simulink model "IM_drive_Simulink"  (R2018b)
settings: Solver=ode45  StartTime=0.0  StopTime=10.0  RelTol=1e-6  AbsTol=1e-8
values from neighbouring files (symbols this model uses):
  AntiW = 1    [IM_drive_main_code.m]
  B = 0.08    [IM_drive_main_code.m]
  Ba = (alfaw*Jhat-Bhat)*1    (= 0.17)    [IM_drive_main_code.m]
  Flux_ref = 0.9    [IM_drive_main_code.m]
  Flux_ref_time = 0.001    [IM_drive_main_code.m]
  invL_matrix = inv(LMAT)    [IM_drive_main_code.m]
  ir_alpha_0 = 0    [IM_drive_main_code.m]
  ir_beta_0 = 0    [IM_drive_main_code.m]
  is_alpha_0 = 0    [IM_drive_main_code.m]
  is_beta_0 = 0    [IM_drive_main_code.m]
  Israted = 9.1*sqrt(2)    [IM_drive_main_code.m]
  J = 0.0125    [IM_drive_main_code.m]
  Kic = alfac*(Rshat+RRhat+Ra)    (= 15552.4475524)    [IM_drive_main_code.m]
  Kiw = alfaw*(Bhat+Ba)    (= 5)    [IM_drive_main_code.m]
  Kpc = alfac*Lsigmahat    (= 15.5524475524)    [IM_drive_main_code.m]
  Kpw = alfaw*Jhat    (= 0.25)    [IM_drive_main_code.m]
  Lm = 0.135    [IM_drive_main_code.m]
  LMhat = LM*0.9    (= 0.114702797203)    [IM_drive_main_code.m]
  Lr = Lm+Lrl    (= 0.143)    [IM_drive_main_code.m]
  Lsigmahat = Lsigma*1    (= 0.0155524475524)    [IM_drive_main_code.m]
  np = 2    [IM_drive_main_code.m]
  PsiRhat0 = 0    [IM_drive_main_code.m]
  Ra = (alfac*Lsigmahat-Rshat-RRhat)*1    (= 13.1173079368)    [IM_drive_main_code.m]
  RR = (Lm/Lr)^2*Rr    (= 1.10513961563)    [IM_drive_main_code.m]
  Rr = 1.24    [IM_drive_main_code.m]
  RRhat = RR*1    (= 1.10513961563)    [IM_drive_main_code.m]
  Rs = 1.33    [IM_drive_main_code.m]
  Te_ref1 = 12    [IM_drive_main_code.m]
  Te_ref2 = 8    [IM_drive_main_code.m]
  Te_reftime1 = 1    [IM_drive_main_code.m]
  Te_reftime2 = 2    [IM_drive_main_code.m]
  Te_reftime3 = 2.1    [IM_drive_main_code.m]
  thetahat0 = 0    [IM_drive_main_code.m]
  thetar_0 = 0    [IM_drive_main_code.m]
  TL_extra = 14.6    [IM_drive_main_code.m]
  TL_extra_time = 10    [IM_drive_main_code.m]
  Umax = VconvLim    [IM_drive_main_code.m]
  VconvLim = 440*sqrt(2/3)    [IM_drive_main_code.m]
  wr_0 = 0    [IM_drive_main_code.m]
  Wr_ref_step = 1435*pi/30    (= 150.272848597)    [IM_drive_main_code.m]
  Wr_ref_step_time = 1.0    (= 1)    [IM_drive_main_code.m]
undefined symbols (not defined in the file or in its folder): j
settings Model: ExtModeTrigMode=oneshot  ExtModeArmWhenConnect=off  ExtModeAutoUpdateStatusClock=off  Creator=e6zebra  LastModifiedBy=e6zebra
settings SolverCC: AutoScaleAbsTol=off
settings DataIOCC: SaveFormat=Array  SignalLoggingSaveFormat=ModelDataLogs
settings OptimizationCC: BlockReduction=off  BooleanDataType=off  ExpressionDepthLimit=2147483647  InitFltsAndDblsToZero=on  LifeSpan=inf
settings DebuggingCC: SaveWithParameterizedLinksMsg=none  UnderspecifiedInitializationDetection=Classic  MergeDetectMultiDrivingBlocksExec=none  SignalResolutionControl=TryResolveAllWithWarning  MultiTaskDSMMsg=warning  MultiTaskCondExecSysMsg=none  FcnCallInpInsideContextMsg=warning  StateNameClashWarn=warning  SFUnexpectedBacktrackingDiag=warning  SFNoUnconditionalDefaultTransitionDiag=warning  SFExecutionAtInitializationDiag=none
settings HardwareCC: ProdBitPerPointer=32  ProdBitPerSizeT=32  ProdBitPerPtrDiffT=32  ProdLargestAtomicFloat=None  ProdIntDivRoundTo=Undefined  ProdEndianess=Unspecified  ProdWordSize=32  ProdHWDeviceType=32-bit Generic  TargetUnknown=on
settings ModelReferenceCC: PropagateSignalLabelsOutOfModel=off
settings SFSimCC: SimUseLocalCustomCode=off
settings RTWCC: TemplateMakefile=grt.tmf  RTWUseLocalCustomCode=off
settings CodeAppCC: StateflowObjectComments=on
settings GRTTargetCC: TargetFcnLib=ansi_tfl_tmw.mat  TargetLangStandard=C89/C90 (ANSI)  GeneratePreprocessorConditionals=Disable all  CombineOutputUpdateFcns=off  GRTInterface=on
settings ConfigComp: CovMetricSettings=dw  CovHtmlReporting=on  CovSaveCumulativeToWorkspaceVar=on  CovSaveSingleToWorkspaceVar=on  CovExternalEMLEnable=off

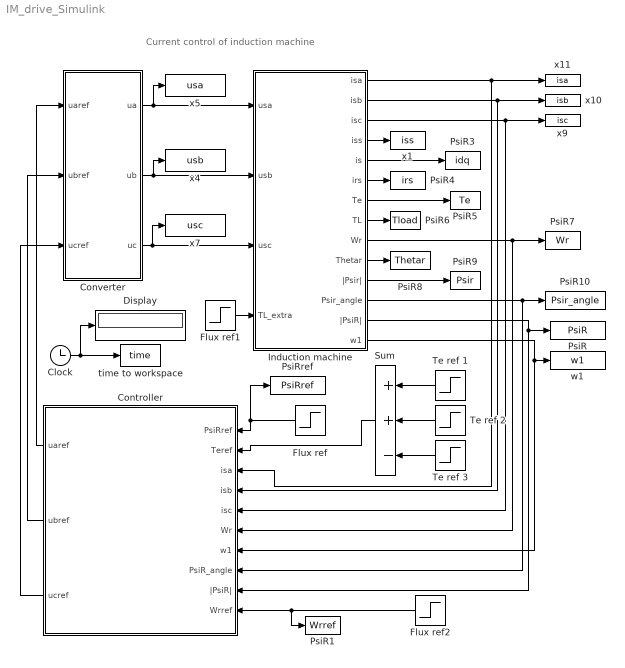
== system IM_drive_Simulink ==
  note: Current control of induction machine
  Clock : Clock
  Controller : Subsystem
  Converter : Subsystem
  Display : Display
  Flux ref : Step  Time=Flux_ref_time  After=Flux_ref  SampleTime=0
  Flux ref1 : Step  Time=TL_extra_time  After=TL_extra  SampleTime=0
  Flux ref2 : Step  Time=Wr_ref_step_time  After=Wr_ref_step  SampleTime=0
  Induction machine : Subsystem
  PsiR : ToWorkspace  VariableName=PsiR  SampleTime=-1
  PsiR1 : ToWorkspace  VariableName=Wrref  SampleTime=-1
  PsiR10 : ToWorkspace  VariableName=Psir_angle  SampleTime=-1
  PsiR3 : ToWorkspace  VariableName=idq  SampleTime=-1
  PsiR4 : ToWorkspace  VariableName=irs  SampleTime=-1
  PsiR5 : ToWorkspace  VariableName=Te  SampleTime=-1
  PsiR6 : ToWorkspace  VariableName=Tload  SampleTime=-1
  PsiR7 : ToWorkspace  VariableName=Wr  SampleTime=-1
  PsiR8 : ToWorkspace  VariableName=Thetar  SampleTime=-1
  PsiR9 : ToWorkspace  VariableName=Psir  SampleTime=-1
  PsiRref : ToWorkspace  VariableName=PsiRref  SampleTime=-1
  Sum : Sum  Inputs=++-  SaturateOnIntegerOverflow=on
  Te ref 1 : Step  Time=Te_reftime1  After=Te_ref1  SampleTime=0
  Te ref 2 : Step  Time=Te_reftime2  After=Te_ref2  SampleTime=0
  Te ref 3 : Step  Time=Te_reftime3  After=Te_ref2  SampleTime=0
  time to workspace : ToWorkspace  VariableName=time  SampleTime=-1
  w1 : ToWorkspace  VariableName=w1  SampleTime=-1
  x1 : ToWorkspace  VariableName=iss  SampleTime=-1
  x10 : ToWorkspace  VariableName=isb  SampleTime=-1
  x11 : ToWorkspace  VariableName=isa  SampleTime=-1
  x4 : ToWorkspace  VariableName=usb  SampleTime=-1
  x5 : ToWorkspace  VariableName=usa  SampleTime=-1
  x7 : ToWorkspace  VariableName=usc  SampleTime=-1
  x9 : ToWorkspace  VariableName=isc  SampleTime=-1
  wires:
  Clock/1 -> time to workspace/1, Display/1
  Te ref 1/1 -> Sum/1
  Te ref 3/1 -> Sum/3
  Te ref 2/1 -> Sum/2
  Converter/1(ua) -> Induction machine/1(usa), x5/1
  Converter/2(ub) -> Induction machine/2(usb), x4/1
  Converter/3(uc) -> x7/1, Induction machine/3(usc)
  Induction machine/4(iss) -> x1/1
  Induction machine/5(is) -> PsiR3/1
  Induction machine/7(Te) -> PsiR5/1
  Induction machine/6(irs) -> PsiR4/1
  Induction machine/9(Wr) -> Controller/6(Wr), PsiR7/1
  Induction machine/8(TL) -> PsiR6/1
  Induction machine/11(|Psir|) -> PsiR9/1
  Induction machine/10(Thetar) -> PsiR8/1
  Induction machine/12(Psir_angle) -> PsiR10/1, Controller/8(PsiR_angle)
  Induction machine/3(isc) -> Controller/5(isc), x9/1
  Induction machine/2(isb) -> Controller/4(isb), x10/1
  Induction machine/1(isa) -> x11/1, Controller/3(isa)
  Flux ref1/1 -> Induction machine/4(TL_extra)
  Induction machine/13(|PsiR|) -> Controller/9(|PsiR|), PsiR/1
  Induction machine/14(w1) -> Controller/7(w1), w1/1
  Flux ref/1 -> Controller/1(PsiRref), PsiRref/1
  Sum/1 -> Controller/2(Teref)
  Controller/1(uaref) -> Converter/1(uaref)
  Controller/2(ubref) -> Converter/2(ubref)
  Controller/3(ucref) -> Converter/3(ucref)
  Flux ref2/1 -> PsiR1/1, Controller/10(Wrref)

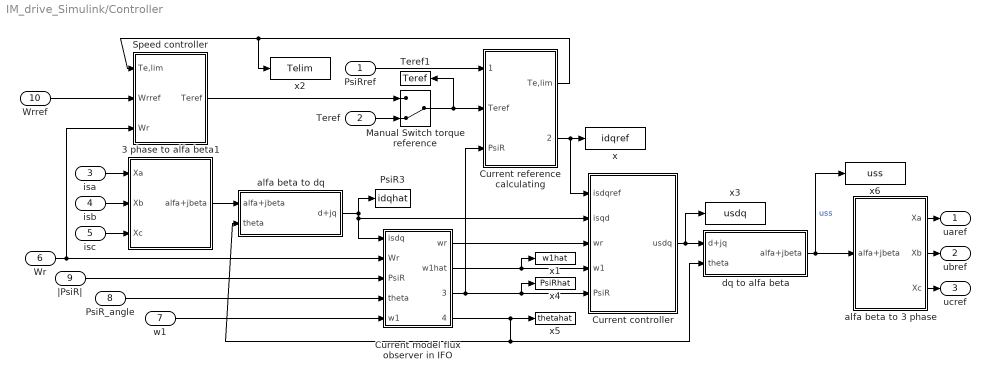
== system IM_drive_Simulink/Controller ==
  PsiRref : Inport
  Teref : Inport  Port=2
  isa : Inport  Port=3
  isb : Inport  Port=4
  isc : Inport  Port=5
  Wr : Inport  Port=6
  w1 : Inport  Port=7
  PsiR_angle : Inport  Port=8
  |PsiR| : Inport  Port=9
  Wrref : Inport  Port=10
  3 phase to alfa beta1 : Subsystem
  Current controller : Subsystem
  Current model flux observer in IFO : Subsystem
  Current reference calculating : Subsystem
  Manual Switch torque reference : ManualSwitch  CurrentSetting=0
  PsiR3 : ToWorkspace  VariableName=idqhat  SampleTime=-1
  Speed controller : Subsystem
  Teref1 : ToWorkspace  VariableName=Teref  SampleTime=-1
  alfa beta to 3 phase : Subsystem
  alfa beta to dq : Subsystem
  dq to alfa beta : Subsystem
  x : ToWorkspace  VariableName=idqref  SampleTime=-1
  x1 : ToWorkspace  VariableName=w1hat  SampleTime=-1
  x2 : ToWorkspace  VariableName=Telim  SampleTime=-1
  x3 : ToWorkspace  VariableName=usdq  SampleTime=-1
  x4 : ToWorkspace  VariableName=PsiRhat  SampleTime=-1
  x5 : ToWorkspace  VariableName=thetahat  SampleTime=-1
  x6 : ToWorkspace  VariableName=uss  SampleTime=-1
  uaref : Outport
  ubref : Outport  Port=2
  ucref : Outport  Port=3
  wires:
  PsiRref/1 -> Current reference calculating/1(PsiRref)
  alfa beta to 3 phase/1(Xa) -> uaref/1
  alfa beta to 3 phase/2(Xb) -> ubref/1
  alfa beta to 3 phase/3(Xc) -> ucref/1
  Current controller/1(usdq) -> x3/1, dq to alfa beta/1(d+jq)
  Current reference calculating/2(isdqref) -> Current controller/1(isdqref), x/1
  dq to alfa beta/1(alfa+jbeta) -> x6/1, alfa beta to 3 phase/1(alfa+jbeta)  "uss"
  Teref/1 -> Manual Switch torque reference/2
  Wr/1 -> Speed controller/3(Wr), Current model flux observer in IFO/2(Wr)
  alfa beta to dq/1(d+jq) -> Current controller/2(isqd), Current model flux observer in IFO/1(isdq), PsiR3/1
  3 phase to alfa beta1/1(alfa+jbeta) -> alfa beta to dq/1(alfa+jbeta)
  isa/1 -> 3 phase to alfa beta1/1(Xa)
  isc/1 -> 3 phase to alfa beta1/3(Xc)
  isb/1 -> 3 phase to alfa beta1/2(Xb)
  Manual Switch torque reference/1 -> Teref1/1, Current reference calculating/2(Teref)
  Current model flux observer in IFO/1(wr) -> Current controller/3(wr)
  Current model flux observer in IFO/2(w1hat) -> x1/1, Current controller/4(w1)
  Current model flux observer in IFO/3(PsiRhat) -> Current reference calculating/3(PsiR), x4/1, Current controller/5(PsiR)
  Current reference calculating/1(Te,lim) -> x2/1, Speed controller/1(Te,lim)
  Speed controller/1(Teref) -> Manual Switch torque reference/1
  w1/1 -> Current model flux observer in IFO/5(w1)
  |PsiR|/1 -> Current model flux observer in IFO/3(PsiR)
  PsiR_angle/1 -> Current model flux observer in IFO/4(theta)
  Current model flux observer in IFO/4(thetahat) -> dq to alfa beta/2(theta), alfa beta to dq/2(theta), x5/1
  Wrref/1 -> Speed controller/2(Wrref)

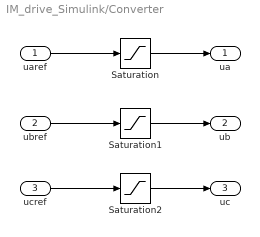
== system IM_drive_Simulink/Converter ==
  uaref : Inport
  ubref : Inport  Port=2
  ucref : Inport  Port=3
  Saturation : Saturate  UpperLimit=VconvLim  LowerLimit=-VconvLim
  Saturation1 : Saturate  UpperLimit=VconvLim  LowerLimit=-VconvLim
  Saturation2 : Saturate  UpperLimit=VconvLim  LowerLimit=-VconvLim
  ua : Outport
  ub : Outport  Port=2
  uc : Outport  Port=3
  wires:
  Saturation2/1 -> uc/1
  Saturation1/1 -> ub/1
  Saturation/1 -> ua/1
  uaref/1 -> Saturation/1
  ubref/1 -> Saturation1/1
  ucref/1 -> Saturation2/1

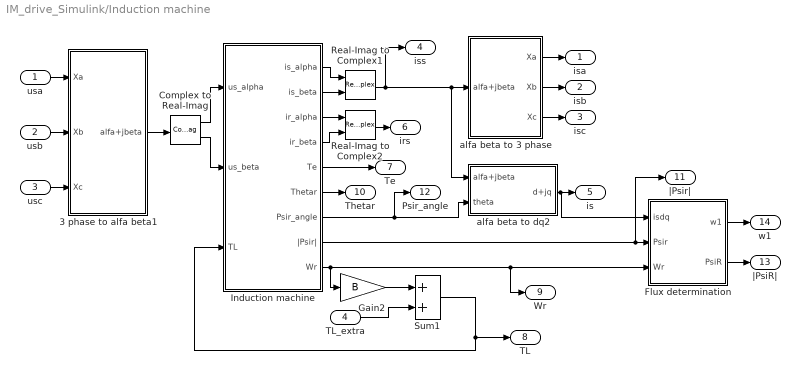
== system IM_drive_Simulink/Induction machine ==
  usa : Inport
  usb : Inport  Port=2
  usc : Inport  Port=3
  TL_extra : Inport  Port=4
  3 phase to alfa beta1 : Subsystem
  Complex to Real-Imag : ComplexToRealImag
  Flux determination : Subsystem
  Gain2 : Gain  Gain=B
  Induction machine : Subsystem
  Real-Imag to Complex1 : RealImagToComplex
  Real-Imag to Complex2 : RealImagToComplex
  Sum1 : Sum  SaturateOnIntegerOverflow=on  InputSameDT=on  OutDataTypeStr=Inherit: Same as first input
  alfa beta to 3 phase : Subsystem
  alfa beta to dq2 : Subsystem
  isa : Outport
  isb : Outport  Port=2
  isc : Outport  Port=3
  iss : Outport  Port=4
  is : Outport  Port=5
  irs : Outport  Port=6
  Te : Outport  Port=7
  TL : Outport  Port=8
  Wr : Outport  Port=9
  Thetar : Outport  Port=10
  |Psir| : Outport  Port=11
  Psir_angle : Outport  Port=12
  |PsiR| : Outport  Port=13
  w1 : Outport  Port=14
  wires:
  TL_extra/1 -> Sum1/2
  Real-Imag to Complex1/1 -> iss/1, alfa beta to 3 phase/1(alfa+jbeta), alfa beta to dq2/1(alfa+jbeta)
  alfa beta to dq2/1(d+jq) -> Flux determination/1(isdq), is/1
  Real-Imag to Complex2/1 -> irs/1
  Sum1/1 -> Induction machine/3(TL), TL/1
  Gain2/1 -> Sum1/1
  3 phase to alfa beta1/1(alfa+jbeta) -> Complex to Real-Imag/1
  usc/1 -> 3 phase to alfa beta1/3(Xc)
  usb/1 -> 3 phase to alfa beta1/2(Xb)
  usa/1 -> 3 phase to alfa beta1/1(Xa)
  alfa beta to 3 phase/1(Xa) -> isa/1
  alfa beta to 3 phase/3(Xc) -> isc/1
  alfa beta to 3 phase/2(Xb) -> isb/1
  Flux determination/2(PsiR) -> |PsiR|/1
  Flux determination/1(w1) -> w1/1
  Induction machine/7(Psir_angle) -> alfa beta to dq2/2(theta), Psir_angle/1
  Induction machine/9(Wr) -> Wr/1, Flux determination/3(Wr), Gain2/1
  Complex to Real-Imag/1 -> Induction machine/1(us_alpha)
  Complex to Real-Imag/2 -> Induction machine/2(us_beta)
  Induction machine/1(is_alpha) -> Real-Imag to Complex1/1
  Induction machine/2(is_beta) -> Real-Imag to Complex1/2
  Induction machine/3(ir_alpha) -> Real-Imag to Complex2/1
  Induction machine/4(ir_beta) -> Real-Imag to Complex2/2
  Induction machine/5(Te) -> Te/1
  Induction machine/6(Thetar) -> Thetar/1
  Induction machine/8(|Psir|) -> |Psir|/1, Flux determination/2(Psir)

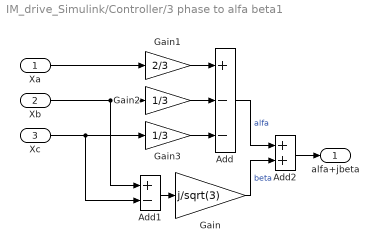
== system IM_drive_Simulink/Controller/3 phase to alfa beta1 ==
  Xa : Inport
  Xb : Inport  Port=2
  Xc : Inport  Port=3
  Add : Sum  Inputs=+--
  Add1 : Sum  Inputs=+-
  Add2 : Sum
  Gain : Gain  Gain=j/sqrt(3)
  Gain1 : Gain  Gain=2/3
  Gain2 : Gain  Gain=1/3
  Gain3 : Gain  Gain=1/3
  alfa+jbeta : Outport
  wires:
  Add1/1 -> Gain/1
  Add2/1 -> alfa+jbeta/1
  Gain/1 -> Add2/2  "beta"
  Add/1 -> Add2/1  "alfa"
  Gain3/1 -> Add/3
  Gain2/1 -> Add/2
  Gain1/1 -> Add/1
  Xa/1 -> Gain1/1
  Xb/1 -> Gain2/1, Add1/1
  Xc/1 -> Gain3/1, Add1/2

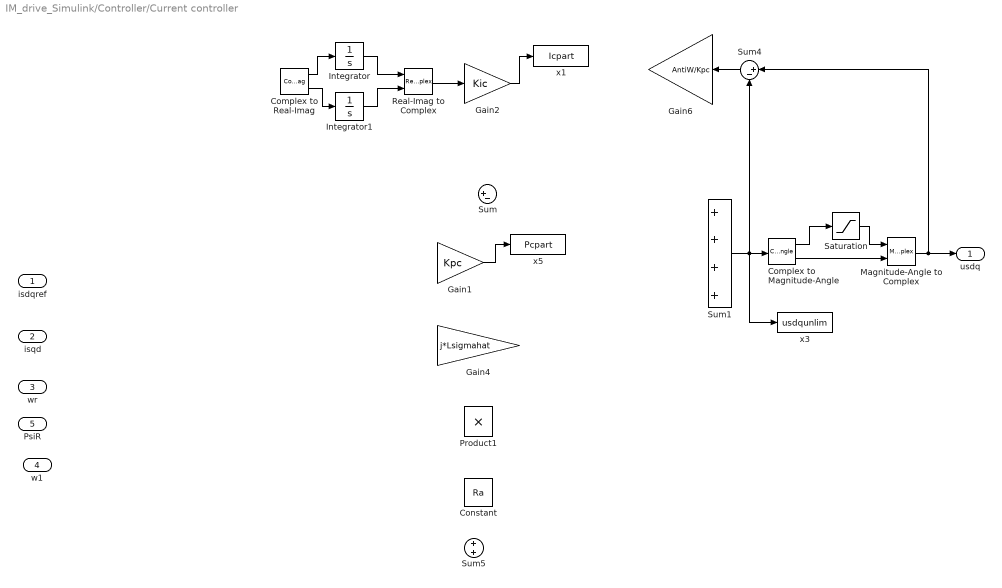
== system IM_drive_Simulink/Controller/Current controller ==
  isdqref : Inport
  isqd : Inport  Port=2
  wr : Inport  Port=3
  w1 : Inport  Port=4
  PsiR : Inport  Port=5
  Complex to Magnitude-Angle : ComplexToMagnitudeAngle
  Complex to Real-Imag : ComplexToRealImag
  Constant : Constant  Value=Ra
  Gain1 : Gain  Gain=Kpc  SaturateOnIntegerOverflow=on  OutDataTypeStr=Inherit: Same as input  ParamDataTypeStr=Inherit: Same as input
  Gain2 : Gain  Gain=Kic  SaturateOnIntegerOverflow=on  OutDataTypeStr=Inherit: Same as input  ParamDataTypeStr=Inherit: Same as input
  Gain4 : Gain  Gain=j*Lsigmahat  SaturateOnIntegerOverflow=on  OutDataTypeStr=Inherit: Same as input  ParamDataTypeStr=Inherit: Same as input
  Gain6 : Gain  Gain=AntiW/Kpc  SaturateOnIntegerOverflow=on  OutDataTypeStr=Inherit: Same as input  ParamDataTypeStr=Inherit: Same as input
  Integrator : Integrator
  Integrator1 : Integrator
  Magnitude-Angle to Complex : MagnitudeAngleToComplex
  Product1 : Product  SaturateOnIntegerOverflow=on  OutDataTypeStr=Inherit: Same as first input
  Real-Imag to Complex : RealImagToComplex
  Saturation : Saturate  UpperLimit=Umax  LowerLimit=-Umax
  Sum : Sum  Inputs=|+-  SaturateOnIntegerOverflow=on
  Sum1 : Sum  Inputs=++++  SaturateOnIntegerOverflow=on
  Sum4 : Sum  Inputs=|+-  SaturateOnIntegerOverflow=on
  Sum5 : Sum  SaturateOnIntegerOverflow=on
  x1 : ToWorkspace  VariableName=Icpart  SampleTime=-1
  x3 : ToWorkspace  VariableName=usdqunlim  SampleTime=-1
  x5 : ToWorkspace  VariableName=Pcpart  SampleTime=-1
  usdq : Outport
  wires:
  Gain1/1 -> x5/1
  Sum1/1 -> Complex to Magnitude-Angle/1, Sum4/2, x3/1
  Complex to Magnitude-Angle/1 -> Saturation/1
  Saturation/1 -> Magnitude-Angle to Complex/1
  Complex to Magnitude-Angle/2 -> Magnitude-Angle to Complex/2
  Magnitude-Angle to Complex/1 -> usdq/1, Sum4/1
  Complex to Real-Imag/2 -> Integrator1/1
  Complex to Real-Imag/1 -> Integrator/1
  Integrator/1 -> Real-Imag to Complex/1
  Integrator1/1 -> Real-Imag to Complex/2
  Real-Imag to Complex/1 -> Gain2/1
  Gain2/1 -> x1/1
  Sum4/1 -> Gain6/1

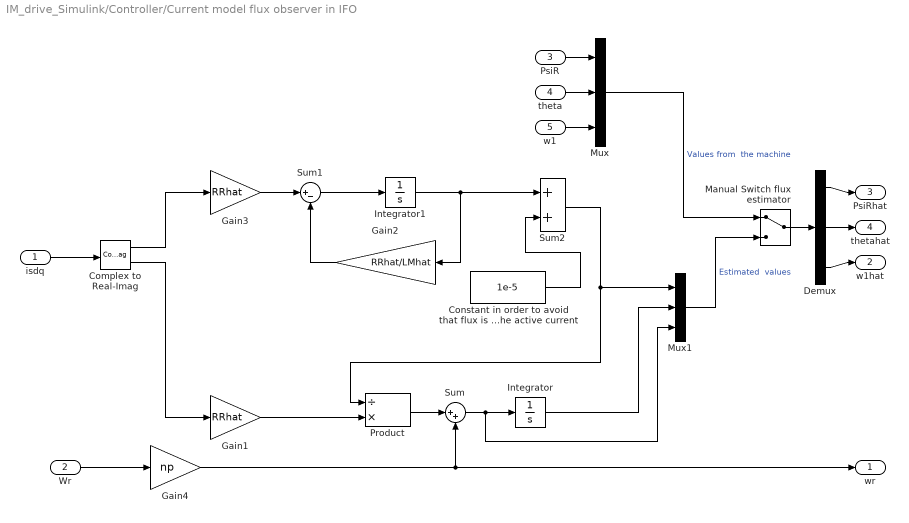
== system IM_drive_Simulink/Controller/Current model flux observer in IFO ==
  isdq : Inport
  Wr : Inport  Port=2
  PsiR : Inport  Port=3
  theta : Inport  Port=4
  w1 : Inport  Port=5
  Complex to Real-Imag : ComplexToRealImag
  "Constant in order to avoid that flux is equal to zero, which will give problems later when deriving the reference value for the active current" : Constant  Value=1e-5
  Demux : Demux  Outputs=3
  Gain1 : Gain  Gain=RRhat  SaturateOnIntegerOverflow=on  OutDataTypeStr=Inherit: Same as input  ParamDataTypeStr=Inherit: Same as input
  Gain2 : Gain  Gain=RRhat/LMhat  SaturateOnIntegerOverflow=on  OutDataTypeStr=Inherit: Same as input  ParamDataTypeStr=Inherit: Same as input
  Gain3 : Gain  Gain=RRhat  SaturateOnIntegerOverflow=on  OutDataTypeStr=Inherit: Same as input  ParamDataTypeStr=Inherit: Same as input
  Gain4 : Gain  Gain=np  SaturateOnIntegerOverflow=on  OutDataTypeStr=Inherit: Same as input  ParamDataTypeStr=Inherit: Same as input
  Integrator : Integrator  InitialCondition=thetahat0
  Integrator1 : Integrator  InitialCondition=PsiRhat0
  Manual Switch flux estimator : ManualSwitch
  Mux : Mux  Inputs=3
  Mux1 : Mux  Inputs=3
  Product : Product  Inputs=/*  SaturateOnIntegerOverflow=on  OutDataTypeStr=Inherit: Same as first input
  Sum : Sum  Inputs=|++  SaturateOnIntegerOverflow=on
  Sum1 : Sum  Inputs=|+-  SaturateOnIntegerOverflow=on
  Sum2 : Sum  SaturateOnIntegerOverflow=on  InputSameDT=on  OutDataTypeStr=Inherit: Same as first input
  wr : Outport
  w1hat : Outport  Port=2
  PsiRhat : Outport  Port=3
  thetahat : Outport  Port=4
  wires:
  Gain1/1 -> Product/2
  Product/1 -> Sum/1
  Wr/1 -> Gain4/1
  Sum/1 -> Mux1/3, Integrator/1
  Integrator/1 -> Mux1/2
  isdq/1 -> Complex to Real-Imag/1
  Complex to Real-Imag/2 -> Gain1/1
  Complex to Real-Imag/1 -> Gain3/1
  Gain3/1 -> Sum1/1
  Sum1/1 -> Integrator1/1
  Integrator1/1 -> Gain2/1, Sum2/1
  Gain2/1 -> Sum1/2
  Sum2/1 -> Mux1/1, Product/1
  "Constant in order to avoid that flux is equal to zero, which will give problems later when deriving the reference value for the active current"/1 -> Sum2/2
  Gain4/1 -> Sum/2, wr/1
  Manual Switch flux estimator/1 -> Demux/1
  Demux/1 -> PsiRhat/1
  Demux/2 -> thetahat/1
  Demux/3 -> w1hat/1
  w1/1 -> Mux/3
  theta/1 -> Mux/2
  PsiR/1 -> Mux/1
  Mux/1 -> Manual Switch flux estimator/1  "Values from  the machine"
  Mux1/1 -> Manual Switch flux estimator/2  "Estimated  values"

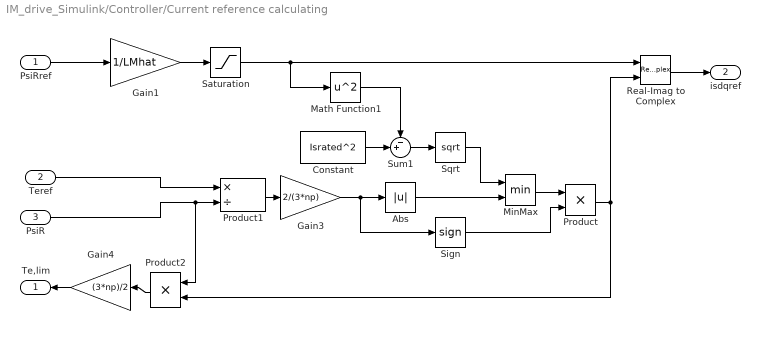
== system IM_drive_Simulink/Controller/Current reference calculating ==
  PsiRref : Inport
  Teref : Inport  Port=2
  PsiR : Inport  Port=3
  Abs : Abs
  Constant : Constant  Value=Israted^2  SampleTime=-1
  Gain1 : Gain  Gain=1/LMhat  SaturateOnIntegerOverflow=on  OutDataTypeStr=Inherit: Same as input  ParamDataTypeStr=Inherit: Same as input
  Gain3 : Gain  Gain=2/(3*np)  SaturateOnIntegerOverflow=on  OutDataTypeStr=Inherit: Same as input  ParamDataTypeStr=Inherit: Same as input
  Gain4 : Gain  Gain=(3*np)/2  SaturateOnIntegerOverflow=on  OutDataTypeStr=Inherit: Same as input  ParamDataTypeStr=Inherit: Same as input
  Math Function1 : Math  Operator=square  SaturateOnIntegerOverflow=on
  MinMax : MinMax  Inputs=2
  Product : Product  RndMeth=Zero
  Product1 : Product  Inputs=*/  SaturateOnIntegerOverflow=on  OutDataTypeStr=Inherit: Same as first input
  Product2 : Product  Inputs=**  SaturateOnIntegerOverflow=on  OutDataTypeStr=Inherit: Same as first input
  Real-Imag to Complex : RealImagToComplex
  Saturation : Saturate  UpperLimit=Israted  LowerLimit=0
  Sign : Signum
  Sqrt : Sqrt  SaturateOnIntegerOverflow=on
  Sum1 : Sum  Inputs=-+|  SaturateOnIntegerOverflow=on
  Te,lim : Outport
  isdqref : Outport  Port=2
  wires:
  Gain4/1 -> Te,lim/1
  PsiR/1 -> Product1/2, Product2/1
  PsiRref/1 -> Gain1/1
  Sign/1 -> Product/2
  MinMax/1 -> Product/1
  Product/1 -> Real-Imag to Complex/2, Product2/2
  Product2/1 -> Gain4/1
  Sqrt/1 -> MinMax/1
  Math Function1/1 -> Sum1/1
  Constant/1 -> Sum1/2
  Teref/1 -> Product1/1
  Abs/1 -> MinMax/2
  Saturation/1 -> Real-Imag to Complex/1, Math Function1/1
  Sum1/1 -> Sqrt/1
  Product1/1 -> Gain3/1
  Real-Imag to Complex/1 -> isdqref/1
  Gain1/1 -> Saturation/1
  Gain3/1 -> Abs/1, Sign/1

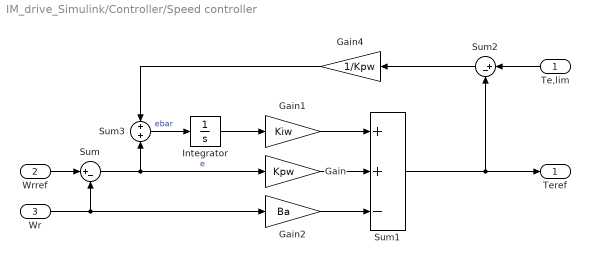
== system IM_drive_Simulink/Controller/Speed controller ==
  Te,lim : Inport
  Wrref : Inport  Port=2
  Wr : Inport  Port=3
  Gain : Gain  Gain=Kpw  SaturateOnIntegerOverflow=on  OutDataTypeStr=Inherit: Same as input  ParamDataTypeStr=Inherit: Same as input
  Gain1 : Gain  Gain=Kiw  SaturateOnIntegerOverflow=on  OutDataTypeStr=Inherit: Same as input  ParamDataTypeStr=Inherit: Same as input
  Gain2 : Gain  Gain=Ba  SaturateOnIntegerOverflow=on  OutDataTypeStr=Inherit: Same as input  ParamDataTypeStr=Inherit: Same as input
  Gain4 : Gain  Gain=1/Kpw  SaturateOnIntegerOverflow=on  OutDataTypeStr=Inherit: Same as input  ParamDataTypeStr=Inherit: Same as input
  Integrator : Integrator
  Sum : Sum  Inputs=|+-  SaturateOnIntegerOverflow=on
  Sum1 : Sum  Inputs=++-  SaturateOnIntegerOverflow=on
  Sum2 : Sum  Inputs=|+-  SaturateOnIntegerOverflow=on
  Sum3 : Sum  SaturateOnIntegerOverflow=on
  Teref : Outport
  wires:
  Gain/1 -> Sum1/2
  Gain1/1 -> Sum1/1
  Integrator/1 -> Gain1/1
  Sum1/1 -> Teref/1, Sum2/2
  Sum/1 -> Gain/1, Sum3/2  "e"
  Sum3/1 -> Integrator/1  "ebar"
  Sum2/1 -> Gain4/1
  Gain4/1 -> Sum3/1
  Gain2/1 -> Sum1/3
  Wrref/1 -> Sum/1
  Wr/1 -> Sum/2, Gain2/1
  Te,lim/1 -> Sum2/1

== system IM_drive_Simulink/Controller/alfa beta to 3 phase ==
  alfa+jbeta : Inport
  Add1 : Sum  Inputs=-+
  Add2 : Sum  Inputs=--
  Complex to Real-Imag : ComplexToRealImag
  Gain1 : Gain  Gain=sqrt(3)/2
  Gain2 : Gain  Gain=1/2
  Xa : Outport
  Xb : Outport  Port=2
  Xc : Outport  Port=3
  wires:
  alfa+jbeta/1 -> Complex to Real-Imag/1
  Complex to Real-Imag/1 -> Xa/1, Gain2/1
  Add2/1 -> Xc/1
  Add1/1 -> Xb/1
  Complex to Real-Imag/2 -> Gain1/1
  Gain1/1 -> Add1/2, Add2/2
  Gain2/1 -> Add1/1, Add2/1

== system IM_drive_Simulink/Controller/alfa beta to dq ==
  alfa+jbeta : Inport
  theta : Inport  Port=2
  Gain : Gain  Gain=-j  SaturateOnIntegerOverflow=on  OutDataTypeStr=Inherit: Same as input  ParamDataTypeStr=Inherit: Same as input
  Math Function : Math  SaturateOnIntegerOverflow=on
  Product : Product  SaturateOnIntegerOverflow=on  OutDataTypeStr=Inherit: Same as first input
  d+jq : Outport
  wires:
  theta/1 -> Gain/1
  Gain/1 -> Math Function/1
  Math Function/1 -> Product/2
  alfa+jbeta/1 -> Product/1
  Product/1 -> d+jq/1

== system IM_drive_Simulink/Controller/dq to alfa beta ==
  d+jq : Inport
  theta : Inport  Port=2
  Gain : Gain  Gain=j  SaturateOnIntegerOverflow=on  OutDataTypeStr=Inherit: Same as input  ParamDataTypeStr=Inherit: Same as input
  Math Function : Math  SaturateOnIntegerOverflow=on
  Product : Product  SaturateOnIntegerOverflow=on  OutDataTypeStr=Inherit: Same as first input
  alfa+jbeta : Outport
  wires:
  theta/1 -> Gain/1
  Gain/1 -> Math Function/1
  Math Function/1 -> Product/2
  d+jq/1 -> Product/1
  Product/1 -> alfa+jbeta/1

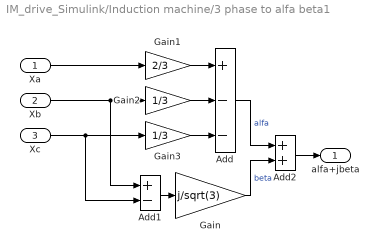
== system IM_drive_Simulink/Induction machine/3 phase to alfa beta1 ==
  Xa : Inport
  Xb : Inport  Port=2
  Xc : Inport  Port=3
  Add : Sum  Inputs=+--
  Add1 : Sum  Inputs=+-
  Add2 : Sum
  Gain : Gain  Gain=j/sqrt(3)
  Gain1 : Gain  Gain=2/3
  Gain2 : Gain  Gain=1/3
  Gain3 : Gain  Gain=1/3
  alfa+jbeta : Outport
  wires:
  Add1/1 -> Gain/1
  Add2/1 -> alfa+jbeta/1
  Gain/1 -> Add2/2  "beta"
  Add/1 -> Add2/1  "alfa"
  Gain3/1 -> Add/3
  Gain2/1 -> Add/2
  Gain1/1 -> Add/1
  Xa/1 -> Gain1/1
  Xb/1 -> Gain2/1, Add1/1
  Xc/1 -> Gain3/1, Add1/2

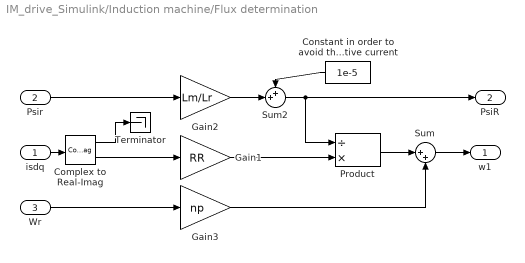
== system IM_drive_Simulink/Induction machine/Flux determination ==
  isdq : Inport
  Psir : Inport  Port=2
  Wr : Inport  Port=3
  Complex to Real-Imag : ComplexToRealImag
  "Constant in order to avoid that flux is equal to zero, which will give problems later when deriving the reference value for the active current" : Constant  Value=1e-5
  Gain1 : Gain  Gain=RR  SaturateOnIntegerOverflow=on  OutDataTypeStr=Inherit: Same as input  ParamDataTypeStr=Inherit: Same as input
  Gain2 : Gain  Gain=Lm/Lr  SaturateOnIntegerOverflow=on  OutDataTypeStr=Inherit: Same as input  ParamDataTypeStr=Inherit: Same as input
  Gain3 : Gain  Gain=np  SaturateOnIntegerOverflow=on  OutDataTypeStr=Inherit: Same as input  ParamDataTypeStr=Inherit: Same as input
  Product : Product  Inputs=/*  SaturateOnIntegerOverflow=on  OutDataTypeStr=Inherit: Same as first input
  Sum : Sum  Inputs=|++  SaturateOnIntegerOverflow=on
  Sum2 : Sum  Inputs=++|  SaturateOnIntegerOverflow=on  InputSameDT=on  OutDataTypeStr=Inherit: Same as first input
  Terminator : Terminator
  w1 : Outport
  PsiR : Outport  Port=2
  wires:
  Gain1/1 -> Product/2
  Product/1 -> Sum/1
  Sum/1 -> w1/1
  Wr/1 -> Gain3/1
  Psir/1 -> Gain2/1
  Sum2/1 -> PsiR/1, Product/1
  Gain3/1 -> Sum/2
  Complex to Real-Imag/1 -> Terminator/1
  isdq/1 -> Complex to Real-Imag/1
  Complex to Real-Imag/2 -> Gain1/1
  "Constant in order to avoid that flux is equal to zero, which will give problems later when deriving the reference value for the active current"/1 -> Sum2/1
  Gain2/1 -> Sum2/2

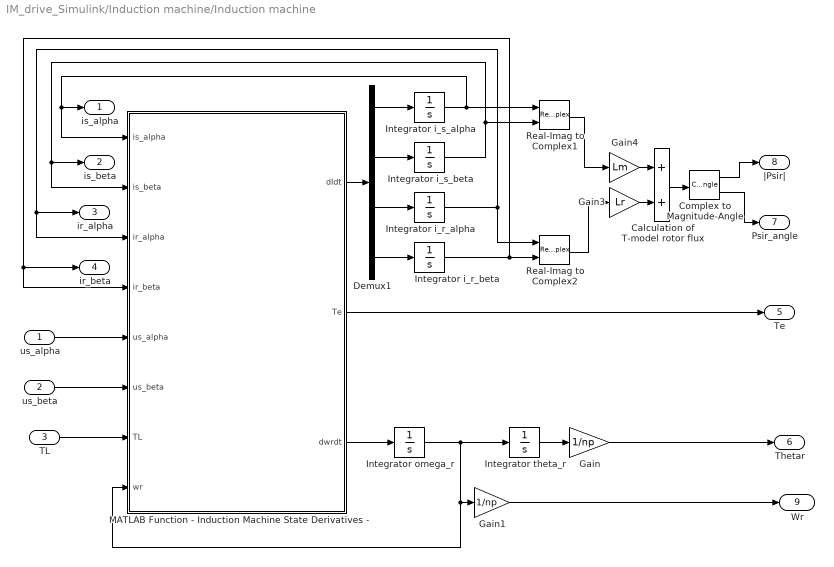
== system IM_drive_Simulink/Induction machine/Induction machine ==
  us_alpha : Inport
  us_beta : Inport  Port=2
  TL : Inport  Port=3
  Calculation of T-model rotor flux : Sum  SaturateOnIntegerOverflow=on  InputSameDT=on  OutDataTypeStr=Inherit: Same as first input
  Complex to Magnitude-Angle : ComplexToMagnitudeAngle
  Demux1 : Demux
  Gain : Gain  Gain=1/np
  Gain1 : Gain  Gain=1/np
  Gain3 : Gain  Gain=Lr
  Gain4 : Gain  Gain=Lm
  Integrator i_r_alpha : Integrator  InitialCondition=ir_alpha_0
  Integrator i_r_beta : Integrator  InitialCondition=ir_beta_0
  Integrator i_s_alpha : Integrator  InitialCondition=is_alpha_0
  Integrator i_s_beta : Integrator  InitialCondition=is_beta_0
  Integrator omega_r : Integrator  InitialCondition=wr_0
  Integrator theta_r : Integrator  InitialCondition=thetar_0
  MATLAB Function - Induction Machine State Derivatives - : MATLAB Function  TreatAsAtomicUnit=on
  Real-Imag to Complex1 : RealImagToComplex
  Real-Imag to Complex2 : RealImagToComplex
  is_alpha : Outport
  is_beta : Outport  Port=2
  ir_alpha : Outport  Port=3
  ir_beta : Outport  Port=4
  Te : Outport  Port=5
  Thetar : Outport  Port=6
  Psir_angle : Outport  Port=7
  |Psir| : Outport  Port=8
  Wr : Outport  Port=9
  wires:
  Complex to Magnitude-Angle/1 -> |Psir|/1
  Gain3/1 -> Calculation of T-model rotor flux/2
  Complex to Magnitude-Angle/2 -> Psir_angle/1
  Demux1/4 -> Integrator i_r_beta/1
  Integrator omega_r/1 -> Integrator theta_r/1, Gain1/1, MATLAB Function - Induction Machine State Derivatives -/8(wr)
  Gain/1 -> Thetar/1
  Integrator i_s_beta/1 -> Real-Imag to Complex1/2, is_beta/1, MATLAB Function - Induction Machine State Derivatives -/2(is_beta)
  Calculation of T-model rotor flux/1 -> Complex to Magnitude-Angle/1
  us_beta/1 -> MATLAB Function - Induction Machine State Derivatives -/6(us_beta)
  Demux1/1 -> Integrator i_s_alpha/1
  Gain1/1 -> Wr/1
  Integrator i_r_beta/1 -> ir_beta/1, MATLAB Function - Induction Machine State Derivatives -/4(ir_beta), Real-Imag to Complex2/2
  Integrator i_r_alpha/1 -> Real-Imag to Complex2/1, ir_alpha/1, MATLAB Function - Induction Machine State Derivatives -/3(ir_alpha)
  MATLAB Function - Induction Machine State Derivatives -/2(Te) -> Te/1
  Real-Imag to Complex2/1 -> Gain3/1
  Demux1/3 -> Integrator i_r_alpha/1
  Integrator i_s_alpha/1 -> Real-Imag to Complex1/1, is_alpha/1, MATLAB Function - Induction Machine State Derivatives -/1(is_alpha)
  Demux1/2 -> Integrator i_s_beta/1
  MATLAB Function - Induction Machine State Derivatives -/3(dwrdt) -> Integrator omega_r/1
  Real-Imag to Complex1/1 -> Gain4/1
  us_alpha/1 -> MATLAB Function - Induction Machine State Derivatives -/5(us_alpha)
  TL/1 -> MATLAB Function - Induction Machine State Derivatives -/7(TL)
  MATLAB Function - Induction Machine State Derivatives -/1(dIdt) -> Demux1/1
  Gain4/1 -> Calculation of T-model rotor flux/1
  Integrator theta_r/1 -> Gain/1

== system IM_drive_Simulink/Induction machine/alfa beta to 3 phase ==
  alfa+jbeta : Inport
  Add1 : Sum  Inputs=-+
  Add2 : Sum  Inputs=--
  Complex to Real-Imag : ComplexToRealImag
  Gain1 : Gain  Gain=sqrt(3)/2
  Gain2 : Gain  Gain=1/2
  Xa : Outport
  Xb : Outport  Port=2
  Xc : Outport  Port=3
  wires:
  alfa+jbeta/1 -> Complex to Real-Imag/1
  Complex to Real-Imag/1 -> Xa/1, Gain2/1
  Add2/1 -> Xc/1
  Add1/1 -> Xb/1
  Complex to Real-Imag/2 -> Gain1/1
  Gain1/1 -> Add1/2, Add2/2
  Gain2/1 -> Add1/1, Add2/1

== system IM_drive_Simulink/Induction machine/alfa beta to dq2 ==
  alfa+jbeta : Inport
  theta : Inport  Port=2
  Gain : Gain  Gain=-j  SaturateOnIntegerOverflow=on  OutDataTypeStr=Inherit: Same as input  ParamDataTypeStr=Inherit: Same as input
  Math Function : Math  SaturateOnIntegerOverflow=on
  Product : Product  SaturateOnIntegerOverflow=on  OutDataTypeStr=Inherit: Same as first input
  d+jq : Outport
  wires:
  theta/1 -> Gain/1
  Gain/1 -> Math Function/1
  Math Function/1 -> Product/2
  alfa+jbeta/1 -> Product/1
  Product/1 -> d+jq/1

== matlab function IM_drive_Simulink/Induction machine/Induction machine/MATLAB Function - Induction Machine State Derivatives - ==
  data: is_alpha input; is_beta input; ir_alpha input; ir_beta input; us_alpha input; us_beta input; TL input; dIdt output size=4; Te output size=1; dwrdt output size=1; wr input; np parameter; Rs parameter; Rr parameter; invL_matrix parameter; Lr parameter; Lm parameter; J parameter
function [ dIdt , Te, dwrdt ] = induction_machine_state_derivatives( is_alpha , is_beta, ir_alpha , ir_beta , us_alpha , us_beta , TL , wr , np , Rs , Rr , invL_matrix , Lr , Lm , J)
% Description
% Standard syntax of funtion in MATLAB:
% funtion [ function_outputs ] =function_name( function_inputs )
% Use the same variable names as given in the inputs and outputs of the function

%%%%%%%%%%%%%%%%%%%%%%%%%%%%%%%%%%%%%%%%
% Calculating the electrical Derivatives

% Defining the resistance matrix RMAT
RMAT=[Rs,0,0,0;
	0,Rs,0,0;
	0,wr*Lm,Rr,wr*Lr;
	-wr*Lm,0,-wr*Lr,Rr];

% Defining the current and voltage vectors
I_vector = [ is_alpha ; is_beta ; ir_alpha ; ir_beta ];
U_vector = [ us_alpha ; us_beta ;        0 ;       0 ];

% Calculating the 4 current derivatives
dIdt = -invL_matrix*RMAT * I_vector + invL_matrix*U_vector;

%%%%%%%%%%%%%%%%%%%%%%%%%%%%%%%%%%%%%%%%
% Calculating the Mechanical Derivatives

% Calculating the electrodynamical torque
Te=3*np/2*Lm*(ir_alpha*is_beta-is_alpha*ir_beta);

%  Calculating the rotor speed derivative  
dwrdt=np/J*(Te-TL);

end
